simulink model "Simulink"  (R2020b)
settings: Solver=FixedStepAuto  StartTime=0.0  StopTime=1  FixedStep=Ts  MaxStep=0.001  RelTol=1e-9  AbsTol=1e-9
values from neighbouring files (symbols this model uses):
  alpha = 1000    [Main.m]
  B = 0    [Main.m]
  eta1_est_0 = 0.8*lamda_m    (= 0.256)    [Main.m]
  eta2_est_0 = 0    [Main.m]
  eta_real = lamda_m*[cos(np*theta_0);sin(np*theta_0)]-Z1_0+L*iab_0+R*Z2_0    [Main.m]
  gamma = 0.1    [Main.m]
  iab_0 = [ia_0;ib_0]    [Main.m]
  Jm = 0.00027    [Main.m]
  Kii = Kpi*R/L    (= 6250)    [Main.m]
  KiPLL = Wn^2    (= 360000)    [Main.m]
  Kiw = Jm*wn^2    [Main.m]
  Kpi = 3*L/Tsi    (= 30)    [Main.m]
  KpPLL = 2*xi*Wn*0.3    (= 72)    [Main.m]
  Kpw = 2*xi*Jm*wn-B    [Main.m]
  L = 0.03    [Main.m]
  lamda_m = 0.3200    (= 0.32)    [Main.m]
  np = 5    [Main.m]
  omega_0 = 0    [Main.m]
  R = 6.25    [Main.m]
  theta_0 = 0    [Main.m]
  TL1 = 0.151    [Main.m]
  Z1_0 = [0;0]    [Main.m]
  Z2_0 = [0;0]    [Main.m]
undefined symbols (not defined in the file or in its folder): magnitude, sigbuilder_block
settings Model: Creator=sokra  LastModifiedBy=sokra
settings SolverCC: AutoScaleAbsTol=off

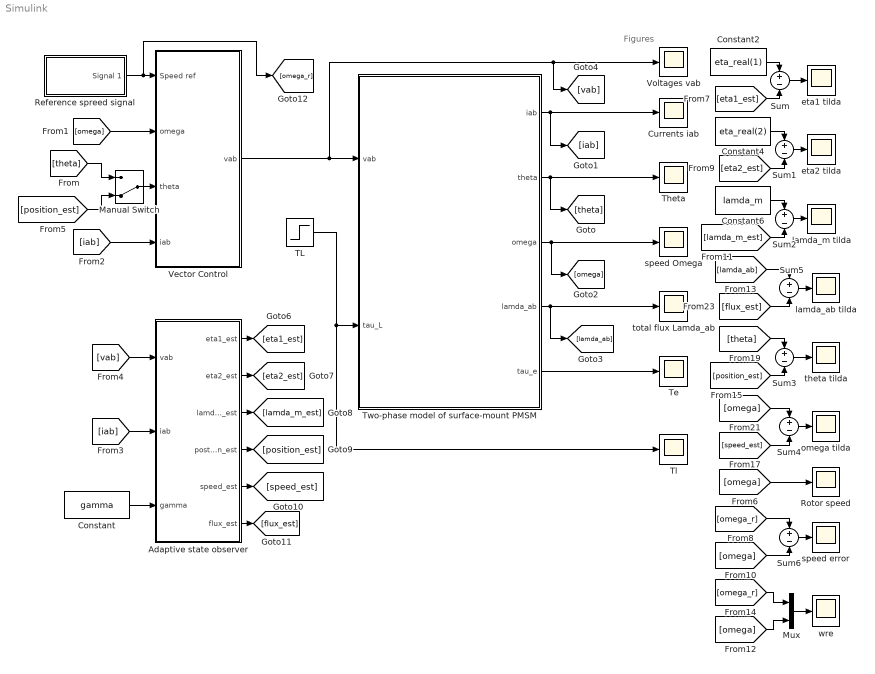
== system Simulink ==
  note: Figures
  Adaptive state observer : Subsystem
  Constant : Constant  Value=gamma
  Constant2 : Constant  Value=eta_real(1)
  Constant4 : Constant  Value=eta_real(2)
  Constant6 : Constant  Value=lamda_m
  Currents iab : Scope
  Manual Switch : ManualSwitch  CurrentSetting=0
  Mux : Mux  Inputs=2
  Reference spreed signal : Subsystem  Tag=STV Subsys  LoadFcn=sigbuilder_block('load');  StartFcn=sigbuilder_block('start');  StopFcn=sigbuilder_block('stop');  ClipboardFcn=sigbuilder_block('clipboard');  mask(Sigbuilder block){tuvar=[0:10]}
      mask help: Simulink:masks:SigbuilderBlock_MD
      mask init:
      | if ~strcmp(get_param(bdroot(gcbh),'SimulationStatus'),'stopped') tuvar = sigbuilder_block('maskInit'); end
      settings: CopyFcn=sigbuilder_block('copy');  DeleteFcn=sigbuilder_block('delete');  ModelCloseFcn=sigbuilder_block('modelClose');  PreSaveFcn=sigbuilder_block('preSave');  PauseFcn=sigbuilder_block('pause');  ContinueFcn=sigbuilder_block('continue');  NameChangeFcn=sigbuilder_block('namechange');  OpenFcn=sigbuilder_block('open',[468 193.5 550.5 318.75 ]);  CloseFcn=sigbuilder_block('close');
      mask Display: plot(0, 0, 100, 100,[2, 2, 32, 32, 2], [68, 8, 8, 68, 68],[32, 2], [38, 38], [32, 19, 2],[53, 60, 44], [32, 17, 17, 2],[16, 16, 31, 31]);txt = getActiveGroup(gcbh);text(2, 100, txt,'verticalAlignment', 'top');
  Rotor speed : Scope
  Sum{,1..6} (7 alike) : Sum  Inputs=+-
  TL : Step  Time=0.5  After=TL1  SampleTime=0
  Te : Scope
  Theta : Scope
  Tl : Scope
  Two-phase model of surface-mount PMSM : Subsystem
  Vector Control : Subsystem
  Voltages vab : Scope
  eta1 tilda : Scope
  eta2 tilda : Scope
  lamda_ab tilda : Scope
  lamda_m tilda : Scope
  omega tilda : Scope
  speed Omega : Scope
  speed error : Scope
  theta tilda : Scope
  total flux Lamda_ab : Scope
  wre : Scope
  wires:
  TL/1 -> Tl/1, Two-phase model of surface-mount PMSM/2(tau_L)
  Two-phase model of surface-mount PMSM/5(tau_e) -> Te/1
  Two-phase model of surface-mount PMSM/4(lamda_ab) -> total flux Lamda_ab/1, [lamda_ab]
  Two-phase model of surface-mount PMSM/1(iab) -> Currents iab/1, [iab]
  Two-phase model of surface-mount PMSM/2(theta) -> Theta/1, [theta]
  Two-phase model of surface-mount PMSM/3(omega) -> speed Omega/1, [omega]
  Vector Control/1(vab) -> Two-phase model of surface-mount PMSM/1(vab), [vab], Voltages vab/1
  Reference spreed signal/1(Signal 1) -> [omega_r], Vector Control/1(Speed ref)
  [omega] -> Vector Control/2(omega)
  [iab] -> Vector Control/4(iab)
  [iab] -> Adaptive state observer/2(iab)
  [vab] -> Adaptive state observer/1(vab)
  Constant/1 -> Adaptive state observer/3(gamma)
  [theta] -> Manual Switch/1
  Manual Switch/1 -> Vector Control/3(theta)
  Adaptive state observer/1(eta1_est) -> [eta1_est]
  Adaptive state observer/3(lamda_m_est) -> [lamda_m_est]
  Adaptive state observer/2(eta2_est) -> [eta2_est]
  Adaptive state observer/4(postion_est) -> [position_est]
  Adaptive state observer/5(speed_est) -> [speed_est]
  Adaptive state observer/6(flux_est) -> [flux_est]
  [position_est] -> Manual Switch/2
  Constant2/1 -> Sum/1
  [eta1_est] -> Sum/2
  Sum/1 -> eta1 tilda/1
  [eta2_est] -> Sum1/2
  Constant4/1 -> Sum1/1
  Sum1/1 -> eta2 tilda/1
  Constant6/1 -> Sum2/1
  [lamda_m_est] -> Sum2/2
  Sum2/1 -> lamda_m tilda/1
  [theta] -> Sum3/1
  [omega] -> Sum4/1
  [speed_est] -> Sum4/2
  Sum4/1 -> omega tilda/1
  Sum5/1 -> lamda_ab tilda/1
  [flux_est] -> Sum5/2
  [lamda_ab] -> Sum5/1
  [position_est] -> Sum3/2
  Sum3/1 -> theta tilda/1
  [omega] -> Rotor speed/1
  Sum6/1 -> speed error/1
  [omega] -> Sum6/2
  [omega_r] -> Sum6/1
  [omega_r] -> Mux/1
  Mux/1 -> wre/1
  [omega] -> Mux/2

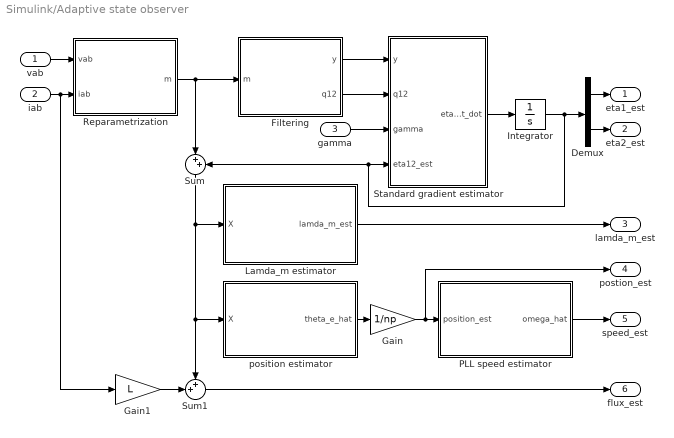
== system Simulink/Adaptive state observer ==
  vab : Inport
  iab : Inport  Port=2
  gamma : Inport  Port=3
  Demux : Demux  Outputs=2
  Filtering : Subsystem
  Gain : Gain  Gain=1/np
  Gain1 : Gain  Gain=L
  Integrator : Integrator  InitialCondition=[eta1_est_0;eta2_est_0]
  Lamda_m estimator : Subsystem
  "PLL speed estimator " : Subsystem
  Reparametrization : Subsystem
  Standard gradient estimator : MATLAB Function  TreatAsAtomicUnit=on
  Sum : Sum  Inputs=|++
  Sum1 : Sum  Inputs=++|
  position estimator : MATLAB Function  TreatAsAtomicUnit=on
  eta1_est : Outport
  eta2_est : Outport  Port=2
  lamda_m_est : Outport  Port=3
  postion_est : Outport  Port=4
  speed_est : Outport  Port=5
  flux_est : Outport  Port=6
  wires:
  iab/1 -> Gain1/1, Reparametrization/2(iab)
  vab/1 -> Reparametrization/1(vab)
  Reparametrization/1(m) -> Sum/1, Filtering/1(m)
  Filtering/1(y) -> Standard gradient estimator/1(y)
  Filtering/2(q12) -> Standard gradient estimator/2(q12)
  gamma/1 -> Standard gradient estimator/3(gamma)
  Standard gradient estimator/1(eta12_est_dot) -> Integrator/1
  Integrator/1 -> Demux/1, Sum/2, Standard gradient estimator/4(eta12_est)
  Demux/1 -> eta1_est/1
  Demux/2 -> eta2_est/1
  Sum/1 -> Sum1/1, position estimator/1(X), Lamda_m estimator/1(X)
  Lamda_m estimator/1(lamda_m_est) -> lamda_m_est/1
  "PLL speed estimator "/1(omega_hat) -> speed_est/1
  position estimator/1(theta_e_hat) -> Gain/1
  Gain/1 -> "PLL speed estimator "/1(position_est), postion_est/1
  Gain1/1 -> Sum1/2
  Sum1/1 -> flux_est/1

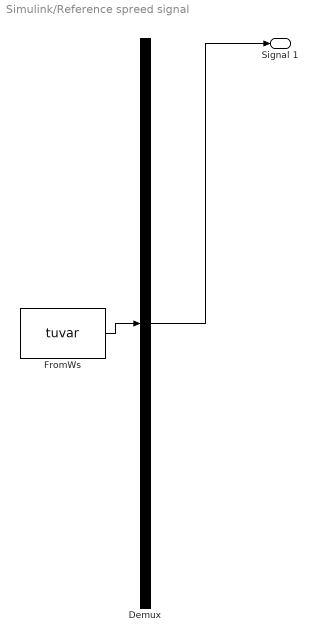
== system Simulink/Reference spreed signal ==
  Demux : Demux  Tag=STV Demux  Outputs=1
      settings: DisplayOption=none
  FromWs : FromWorkspace  Tag=STV FromWs  VariableName=tuvar
      SigBuilderData=|
      | common.afterFinalStr = 'Extrapolate'
      | common.sampleTime = 0
      | dataSet.timeRange = [0 10]
      | dataSet.name = 'Group 1'
      | sbobj.Groups.Name = 'Group 1'
      | sbobj.Groups.Signals.Name = 'Signal 1'
      | sbobj.Groups.Signals.XData = [0 0.2 6 10]
      | sbobj.Groups.Signals.YData = [0 194 194 194]
  Signal 1 : Outport  Tag=STV Outport
  wires:
  Demux/1 -> Signal 1/1
  FromWs/1 -> Demux/1

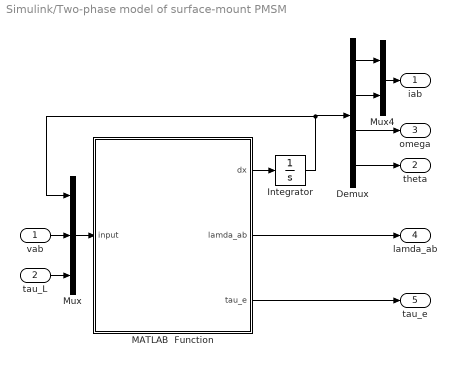
== system Simulink/Two-phase model of surface-mount PMSM ==
  vab : Inport
  tau_L : Inport  Port=2
  Demux : Demux
  Integrator : Integrator  InitialCondition=[iab_0;omega_0;theta_0]
  MATLAB  Function : MATLAB Function  TreatAsAtomicUnit=on
  Mux : Mux  Inputs=3
  Mux4 : Mux  Inputs=2
  iab : Outport
  theta : Outport  Port=2  OutDataTypeStr=double  PortDimensions=1
  omega : Outport  Port=3
  lamda_ab : Outport  Port=4
  tau_e : Outport  Port=5
  wires:
  Mux4/1 -> iab/1
  Mux/1 -> MATLAB  Function/1(input)
  Integrator/1 -> Mux/1, Demux/1
  Demux/2 -> Mux4/2
  vab/1 -> Mux/2
  MATLAB  Function/2(lamda_ab) -> lamda_ab/1
  Demux/1 -> Mux4/1
  tau_L/1 -> Mux/3
  Demux/3 -> omega/1
  Demux/4 -> theta/1
  MATLAB  Function/3(tau_e) -> tau_e/1
  MATLAB  Function/1(dx) -> Integrator/1

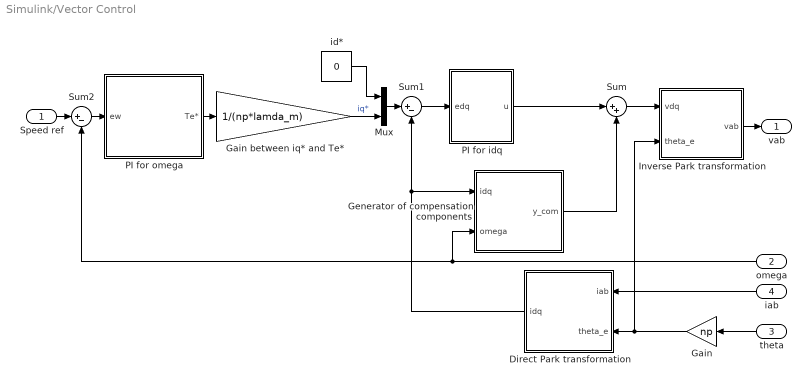
== system Simulink/Vector Control ==
  Speed ref : Inport
  omega : Inport  Port=2
  theta : Inport  Port=3
  iab : Inport  Port=4
  Direct Park transformation : MATLAB Function  TreatAsAtomicUnit=on
  Gain : Gain  Gain=np
  Gain between iq* and Te* : Gain  Gain=1/(np*lamda_m)
  Generator of compensation components : MATLAB Function  TreatAsAtomicUnit=on
  Inverse Park transformation : MATLAB Function  TreatAsAtomicUnit=on
  Mux : Mux  Inputs=2
  PI for idq : Subsystem  mask{Kii_d=Kii, Kpi_d=Kpi, Kii_q=Kii, Kpi_q=Kpi}
  PI for omega : Subsystem  mask{Ki=Kiw, Kp=Kpw}
  Sum : Sum  Inputs=|++
  Sum1 : Sum  Inputs=|+-
  Sum2 : Sum  Inputs=|+-
  id* : Constant  Value=0
  vab : Outport
  wires:
  Generator of compensation components/1(y_com) -> Sum/2
  id*/1 -> Mux/1
  Gain between iq* and Te*/1 -> Mux/2  "iq*"
  Sum/1 -> Inverse Park transformation/1(vdq)
  omega/1 -> Generator of compensation components/2(omega), Sum2/2
  Sum1/1 -> PI for idq/1(edq)
  Mux/1 -> Sum1/1
  Sum2/1 -> PI for omega/1(ew)
  PI for idq/1(u) -> Sum/1
  Gain/1 -> Inverse Park transformation/2(theta_e), Direct Park transformation/2(theta_e)
  PI for omega/1(Te*) -> Gain between iq* and Te*/1
  Direct Park transformation/1(idq) -> Sum1/2, Generator of compensation components/1(idq)
  iab/1 -> Direct Park transformation/1(iab)
  Inverse Park transformation/1(vab) -> vab/1
  Speed ref/1 -> Sum2/1
  theta/1 -> Gain/1

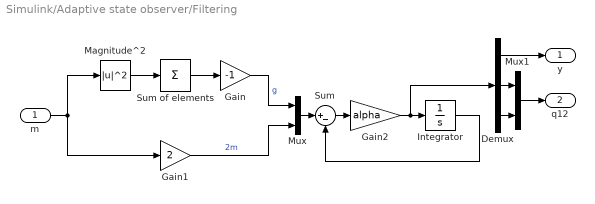
== system Simulink/Adaptive state observer/Filtering ==
  m : Inport
  Demux : Demux  Outputs=3
  Gain : Gain  Gain=-1
  Gain1 : Gain  Gain=2
  Gain2 : Gain  Gain=alpha
  Integrator : Integrator
  Magnitude^2 : Math  Operator=magnitude^2  SaturateOnIntegerOverflow=on
  Mux : Mux  Inputs=2
  Mux1 : Mux  Inputs=2
  Sum : Sum  Inputs=|+-
  Sum of elements : Sum  Inputs=+
  y : Outport
  q12 : Outport  Port=2
  wires:
  Gain/1 -> Mux/1  "g"
  Gain2/1 -> Demux/1, Integrator/1
  Sum of elements/1 -> Gain/1
  m/1 -> Gain1/1, Magnitude^2/1
  Gain1/1 -> Mux/2  "2m"
  Mux/1 -> Sum/1
  Magnitude^2/1 -> Sum of elements/1
  Demux/1 -> y/1
  Sum/1 -> Gain2/1
  Demux/3 -> Mux1/2
  Demux/2 -> Mux1/1
  Mux1/1 -> q12/1
  Integrator/1 -> Sum/2

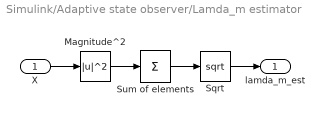
== system Simulink/Adaptive state observer/Lamda_m estimator ==
  X : Inport
  Magnitude^2 : Math  Operator=magnitude^2  SaturateOnIntegerOverflow=on
  Sqrt : Sqrt  SaturateOnIntegerOverflow=on
  Sum of elements : Sum  Inputs=+
  lamda_m_est : Outport
  wires:
  X/1 -> Magnitude^2/1
  Sum of elements/1 -> Sqrt/1
  Magnitude^2/1 -> Sum of elements/1
  Sqrt/1 -> lamda_m_est/1

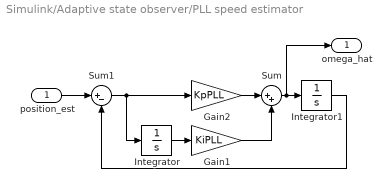
== system Simulink/Adaptive state observer/PLL speed estimator  ==
  position_est : Inport
  Gain1 : Gain  Gain=KiPLL
  Gain2 : Gain  Gain=KpPLL
  Integrator : Integrator
  Integrator1 : Integrator
  Sum : Sum  Inputs=|++
  Sum1 : Sum  Inputs=|+-
  omega_hat : Outport
  wires:
  Sum/1 -> omega_hat/1, Integrator1/1
  Sum1/1 -> Gain2/1, Integrator/1
  Integrator/1 -> Gain1/1
  Gain2/1 -> Sum/1
  Integrator1/1 -> Sum1/2
  position_est/1 -> Sum1/1
  Gain1/1 -> Sum/2

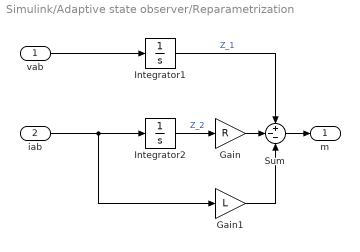
== system Simulink/Adaptive state observer/Reparametrization ==
  vab : Inport
  iab : Inport  Port=2
  Gain : Gain  Gain=R
  Gain1 : Gain  Gain=L
  Integrator1 : Integrator  InitialCondition=Z1_0
  Integrator2 : Integrator  InitialCondition=Z2_0
  Sum : Sum  Inputs=+--
  m : Outport
  wires:
  Integrator2/1 -> Gain/1  "Z_2"
  Sum/1 -> m/1
  Gain/1 -> Sum/2
  iab/1 -> Gain1/1, Integrator2/1
  vab/1 -> Integrator1/1
  Gain1/1 -> Sum/3
  Integrator1/1 -> Sum/1  "Z_1"

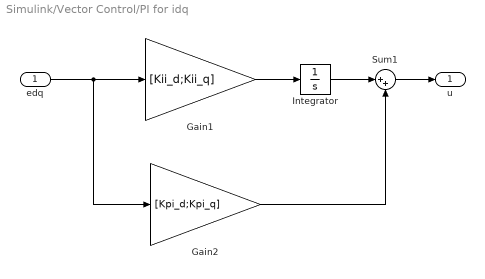
== system Simulink/Vector Control/PI for idq ==
  edq : Inport
  Gain1 : Gain  Gain=[Kii_d;Kii_q]
  Gain2 : Gain  Gain=[Kpi_d;Kpi_q]
  Integrator : Integrator
  Sum1 : Sum  Inputs=|++
  u : Outport
  wires:
  edq/1 -> Gain2/1, Gain1/1
  Gain1/1 -> Integrator/1
  Integrator/1 -> Sum1/1
  Gain2/1 -> Sum1/2
  Sum1/1 -> u/1

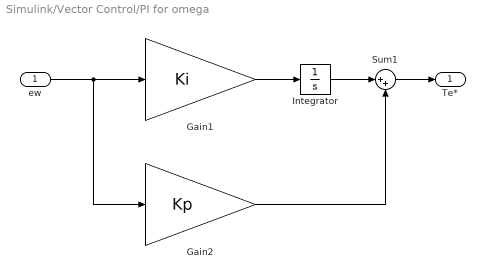
== system Simulink/Vector Control/PI for omega ==
  ew : Inport
  Gain1 : Gain  Gain=Ki
  Gain2 : Gain  Gain=Kp
  Integrator : Integrator
  Sum1 : Sum  Inputs=|++
  Te* : Outport
  wires:
  Sum1/1 -> Te*/1
  Gain2/1 -> Sum1/2
  Integrator/1 -> Sum1/1
  Gain1/1 -> Integrator/1
  ew/1 -> Gain1/1, Gain2/1

== matlab function Simulink/Vector Control/Direct Park transformation ==
  data: iab input; theta_e input; idq output
function idq = fcn(iab,theta_e)
idq = cos(theta_e+[0 -pi/2;pi/2 0])*iab;
end

== matlab function Simulink/Two-phase model of surface-mount PMSM/MATLAB  Function ==
  data: input input; dx output; lamda_ab output; R parameter; L parameter; lamda_m parameter; np parameter; Jm parameter; B parameter; tau_e output
function [dx,lamda_ab,tau_e]  = fcn(input,R, L, lamda_m, np, Jm, B)
ia=input(1);
ib=input(2);
iab=[ia;ib];
omega=input(3);
theta=input(4);
va=input(5);
vb=input(6);
vab=[va;vb];
tau_L=input(7);

%%%%%%%
C=[cos(np*theta);sin(np*theta)];
J=[0 -1;1 0];
dC=np*J*C;
%%%%%%%
dot_iab=(1/L)*(-R*iab-omega*lamda_m*dC+vab);
dot_omega=(1/Jm)*(-B*omega+lamda_m*iab'*dC-tau_L);
dot_theta=omega;
lamda_ab=L*iab+lamda_m*C;
dx = [dot_iab;dot_omega;dot_theta];
tau_e = np * iab' * J * lamda_ab;
end

== matlab function Simulink/Vector Control/Inverse Park transformation ==
  data: vdq input; vab output; theta_e input
function vab = fcn(vdq,theta_e)
vab = cos(theta_e+[0 pi/2;-pi/2 0])*vdq;
end

== matlab function Simulink/Vector Control/Generator of compensation components ==
  data: idq input; omega input; y_com output; np parameter; L parameter; lamda_m parameter
function y_com = fcn(idq,omega,np, L, lamda_m)
y_com=np*omega*[-L*idq(2);(L*idq(1)+lamda_m)];
end

== matlab function Simulink/Adaptive state observer/Standard gradient estimator ==
  data: y input; eta12_est_dot output; q12 input; gamma input; eta12_est input
function eta12_est_dot = fcn(y,q12,gamma,eta12_est)
eta12_est_dot=gamma*q12*(y-q12'*eta12_est);
end

== matlab function Simulink/Adaptive state observer/position estimator ==
  settings: updateMethod=DISCRETE  sampleTime=Ts
  data: X input; theta_e_hat output
function theta_e_hat = fcn(X)

persistent atan2_prev;
if(isempty(atan2_prev))
    atan2_prev=0;
end

persistent theta_e_hat_prev;
if(isempty(theta_e_hat_prev))
    theta_e_hat_prev=0;
end

tan2_now=atan2(X(2),X(1));

Dif=tan2_now-atan2_prev;

if(Dif>pi)
    Dif=Dif-2*pi;
elseif(Dif<(-pi))
    Dif=Dif+2*pi;
end
theta_e_hat=theta_e_hat_prev+Dif;
atan2_prev=tan2_now;
theta_e_hat_prev=theta_e_hat;
end
